simulink model "abs_full_car"  (R2025a)
settings: Solver=ode4  StartTime=0.0  StopTime=6.0  FixedStep=0.0005  RelTol=1e-3
settings Model: Creator=ZORO  LastModifiedBy=ZORO

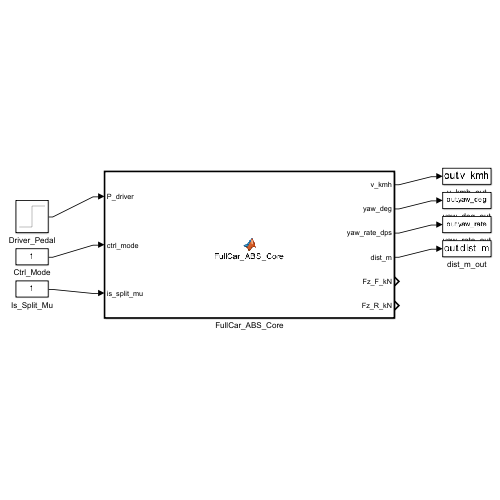
[thumbnail: Simulink's stored preview of the top-level diagram]
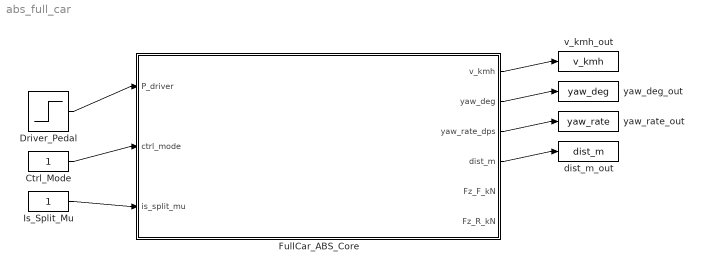
== system abs_full_car ==
  Ctrl_Mode : Constant
  Driver_Pedal : Step  Time=0.10  Before=0.0  After=15.0e6  SampleTime=0
  FullCar_ABS_Core : MATLAB Function  TreatAsAtomicUnit=on
  Is_Split_Mu : Constant
  dist_m_out : ToWorkspace  VariableName=dist_m  SampleTime=-1
  v_kmh_out : ToWorkspace  VariableName=v_kmh  SampleTime=-1
  yaw_deg_out : ToWorkspace  VariableName=yaw_deg  SampleTime=-1
  yaw_rate_out : ToWorkspace  VariableName=yaw_rate  SampleTime=-1
  wires:
  Driver_Pedal/1 -> FullCar_ABS_Core/1(P_driver)
  Ctrl_Mode/1 -> FullCar_ABS_Core/2(ctrl_mode)
  Is_Split_Mu/1 -> FullCar_ABS_Core/3(is_split_mu)
  FullCar_ABS_Core/1(v_kmh) -> v_kmh_out/1
  FullCar_ABS_Core/2(yaw_deg) -> yaw_deg_out/1
  FullCar_ABS_Core/3(yaw_rate_dps) -> yaw_rate_out/1
  FullCar_ABS_Core/4(dist_m) -> dist_m_out/1

== matlab function abs_full_car/FullCar_ABS_Core ==
  data: P_driver input; v_kmh output; ctrl_mode input; is_split_mu input; yaw_deg output; yaw_rate_dps output; dist_m output; Fz_F_kN output; Fz_R_kN output
function [v_kmh, yaw_deg, yaw_rate_dps, dist_m, Fz_F_kN, Fz_R_kN] = FullCar_ABS_Core(P_driver, ctrl_mode, is_split_mu)
% Full Vehicle 4-Wheel ABS Simulation Block
persistent v w x ax psi psi_dot P_act ctrl_phase P_hold w_prev
if isempty(v)
    v = 100 / 3.6;
    w = (v / 0.32) * ones(4, 1);
    x = 0.0;
    ax = 0.0;
    psi = 0.0;
    psi_dot = 0.0;
    P_act = zeros(4, 1);
    ctrl_phase = zeros(4, 1);
    P_hold = zeros(4, 1);
    w_prev = w;
end

dt = 0.0005;
m  = 1600.0;
Jw = 1.20;
R  = 0.32;
L  = 2.60; a = 1.15; b = 1.45;
h  = 0.50; d = 1.55; Iz = 2400.0;
Kb = 1.8e-4;

% Dynamic Pitch Load Transfer
Fz_F_total = max(500.0, (m * 9.81 * b - m * ax * h) / L);
Fz_R_total = max(500.0, (m * 9.81 * a + m * ax * h) / L);
Fz = [Fz_F_total/2; Fz_F_total/2; Fz_R_total/2; Fz_R_total/2];

% Wheel kinematics
vw = w * R;
slip = (v - vw) ./ max(v, 0.1);
slip = max(0.0, min(1.0, slip));

aw = ((w - w_prev) / dt) * R;
w_prev = w;

% Brake command per wheel
P_cmd = zeros(4, 1);
for i = 1:4
    if ctrl_mode == 0 || v < 1.5
        P_cmd(i) = P_driver;
    else
        % Bosch 3-Phase Logic
        is_locking = (slip(i) > 0.19) || (slip(i) > 0.09 && aw(i) < -25.0);
        if ctrl_phase(i) == 0 && is_locking
            ctrl_phase(i) = 2; P_hold(i) = 0.78 * P_act(i);
        elseif ctrl_phase(i) == 2 && (aw(i) > 3.0 || (slip(i) < 0.15 && aw(i) > 0))
            ctrl_phase(i) = 1;
        elseif ctrl_phase(i) == 1 && (aw(i) < 1.5 && slip(i) < 0.14)
            ctrl_phase(i) = 0;
        end
        if ctrl_phase(i) == 2
            P_cmd(i) = max(0.72 * P_hold(i), P_act(i) - 9.0e7 * dt);
        elseif ctrl_phase(i) == 1
            P_cmd(i) = P_hold(i);
        else
            P_cmd(i) = min(P_driver, P_act(i) + 8.5e7 * dt);
        end
    end
end

% Select-Low Yaw Control for split-mu
if is_split_mu > 0 && ctrl_mode > 0
    P_cmd(3) = min(P_cmd(3), P_cmd(4));
    P_cmd(4) = P_cmd(3);
    if abs(P_cmd(1) - P_cmd(2)) > 3.5e6
        if P_cmd(1) > P_cmd(2)
            P_cmd(1) = P_cmd(2) + 3.5e6;
        else
            P_cmd(2) = P_cmd(1) + 3.5e6;
        end
    end
end

% Hydraulic Actuator Dynamics
for i = 1:4
    dP = (P_cmd(i) - P_act(i)) / 0.025;
    dP = max(-1.2e8, min(8.0e7, dP));
    P_act(i) = max(0.0, min(15.0e6, P_act(i) + dP * dt));
end
Tb = Kb * P_act;

% Tire Friction (Split-mu: Left = Dry, Right = Ice)
Fx = zeros(4, 1);
for i = 1:4
    if is_split_mu > 0 && (i == 2 || i == 4)
        B=20.0; C=1.45; D=0.15; E=0.10; % Ice on right wheels
    else
        B=10.0; C=1.60; D=1.00; E=0.40; % Dry asphalt
    end
    arg = B*slip(i) - E*(B*slip(i) - atan(B*slip(i)));
    mu = max(0.0, D * sin(C * atan(arg)));
    Fx(i) = mu * Fz(i);
end

% Yaw Dynamics & Stopping
Mz = ((Fx(1) + Fx(3)) - (Fx(2) + Fx(4))) * (d / 2);
if v > 0.5
    ax = -sum(Fx) / m;
    v  = max(0.0, v + ax * dt);
    x  = x + v * dt;
    psi_dot = psi_dot + (Mz / Iz) * dt;
    psi = psi + psi_dot * dt;
    for i = 1:4
        dw = (-Tb(i) + Fx(i) * R) / Jw;
        w(i) = max(0.0, w(i) + dw * dt);
    end
else
    v = 0.0; w(:) = 0.0; ax = 0.0; psi_dot = 0.0;
end

v_kmh         = v * 3.6;
yaw_deg       = psi * (180 / pi);
yaw_rate_dps  = psi_dot * (180 / pi);
dist_m        = x;
Fz_F_kN       = Fz_F_total * 1e-3;
Fz_R_kN       = Fz_R_total * 1e-3;
